simulink model "prelab5"  (R2023b)
settings: Solver=VariableStepAuto  StartTime=0.0  StopTime=2  RelTol=1e-3
undefined symbols (not defined in the file): magnitude
libraries: dspfdesign x2, commsynccomp2 x1
settings Model: Creator=ASUS  LastModifiedBy=ASUS

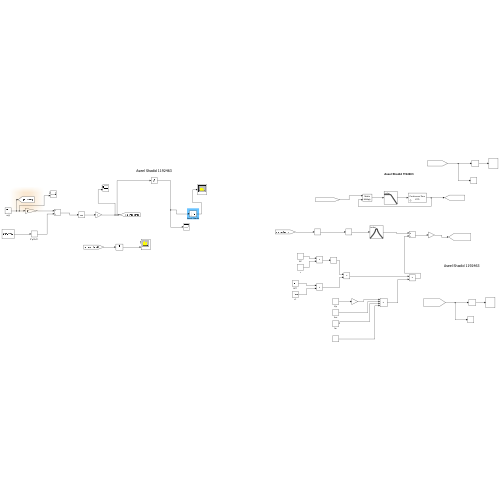
[thumbnail: Simulink's stored preview of the top-level diagram]
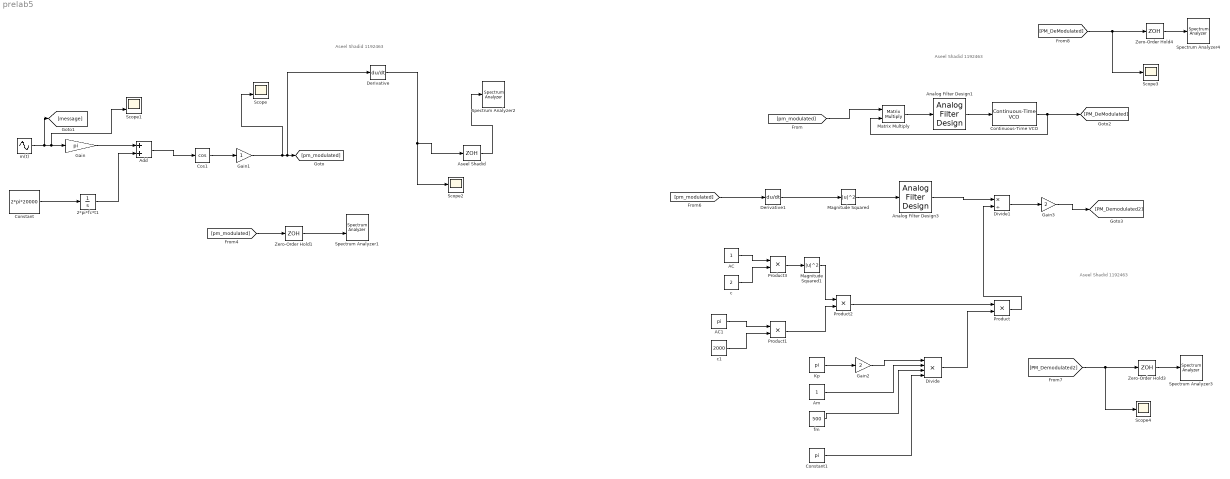
== system prelab5 ==
  note: Aseel Shadid 1192463
  note: Aseel Shadid 1192463
  note: Aseel Shadid 1192463
  " m(t)" : Sin  Frequency=500*pi*2  SampleTime=0
  2*pi*fc*t1 : Integrator
  AC : Constant
  AC1 : Constant  Value=pi
  Add : Sum
  Am : Constant
  Analog Filter Design1 : dspfdesign/Analog Filter Design  method=Butterworth  filttype=Lowpass  N=8  Wlo=pi*2*1000  Whi=80  Rp=2  Rs=40
  Analog Filter Design3 : dspfdesign/Analog Filter Design  method=Butterworth  filttype=Bandpass  N=8  Wlo=pi*2*400  Whi=pi*2*600  Rp=2  Rs=40
  Aseel Shadid : ZeroOrderHold  SampleTime=1/(10*20000)
  Constant : Constant  Value=2*pi*20000
  Constant1 : Constant  Value=pi
  Continuous-Time VCO : commsynccomp2/Continuous-Time VCO  Ac=1  Fc=400  Kc=1  Ph=0
  Cos1 : Trigonometry  Operator=cos
  Derivative : Derivative
  Derivative1 : Derivative
  Divide : Product  Inputs=****
  Divide1 : Product  Inputs=*/
  Gain : Gain  Gain=pi
  Gain1 : Gain
  Gain2 : Gain  Gain=2
  Gain3 : Gain  Gain=2
  Kp : Constant  Value=pi
  Magnitude Squared : Math  Operator=magnitude^2
  Magnitude Squared1 : Math  Operator=magnitude^2
  Matrix Multiply : Product  Multiplication=Matrix(*)
  Product{,1..3} (4 alike) : Product
  Scope : Scope  NumInputPorts=2
  Scope1 : Scope  NumInputPorts=2
  Scope2 : Scope
  Scope3 : Scope
  Scope4 : Scope
  Spectrum Analyzer1 : SpectrumAnalyzer  NumInputPorts=2  WindowPosition=[151.000000,138.000000,1280.000000,605.000000,]  ScopeFrameLocation=window  SpectrumType=RMS  Method=Welch  SampleRate=200000  AxesScaling=Manual  Span=200000  StartFrequency=-100000  StopFrequency=100000  AveragingMethod=Running  SpectrumUnits=Vrms  YLimits=[-0.059214814457474507225,0.53293338124662115174]  DefaultConfigurationName=spbscopes.SpectrumAnalyzerBlockCfg  IsFrequencyInputMode=0  FrequencyVectorPort=0  FrequencyVectorFromPort=0  FrequencyInputRBWPort=0  FrequencyInputRBWFromPort=0
  Spectrum Analyzer2 : SpectrumAnalyzer  WindowPosition=[99.000000,50.000000,1280.000000,605.000000,]  ScopeFrameLocation=window  SpectrumType=RMS  Method=Welch  SampleRate=200000  AxesScaling=Manual  Span=200000  StartFrequency=-100000  StopFrequency=100000  AveragingMethod=Running  SpectrumUnits=Vrms  YLimits=[-3722.990102194120027,33506.911157803537208]  DefaultConfigurationName=spbscopes.SpectrumAnalyzerBlockCfg  IsFrequencyInputMode=0  FrequencyVectorPort=0  FrequencyVectorFromPort=0  FrequencyInputRBWPort=0  FrequencyInputRBWFromPort=0
  Spectrum Analyzer3 : SpectrumAnalyzer  WindowPosition=[15.000000,87.000000,1280.000000,605.000000,]  ScopeFrameLocation=window  SpectrumType=RMS  Method=Welch  SampleRate=200000  AxesScaling=Manual  Span=199999.99999999997  StartFrequency=-99999.99999999999  StopFrequency=99999.99999999999  AveragingMethod=Running  SpectrumUnits=Vrms  YLimits=[-0.54752572772996410677,4.9277315678643134333]  DefaultConfigurationName=spbscopes.SpectrumAnalyzerBlockCfg  IsFrequencyInputMode=0  FrequencyVectorPort=0  FrequencyVectorFromPort=0  FrequencyInputRBWPort=0  FrequencyInputRBWFromPort=0
  Spectrum Analyzer4 : SpectrumAnalyzer  WindowPosition=[-1.000000,139.000000,1280.000000,605.000000,]  ScopeFrameLocation=window  SpectrumType=RMS  Method=Welch  SampleRate=200000  AxesScaling=Manual  Span=200000  StartFrequency=-100000  StopFrequency=100000  AveragingMethod=Running  SpectrumUnits=Vrms  YLimits=[-0.06230515778296413093,0.56074642006213926138]  DefaultConfigurationName=spbscopes.SpectrumAnalyzerBlockCfg  IsFrequencyInputMode=0  FrequencyVectorPort=0  FrequencyVectorFromPort=0  FrequencyInputRBWPort=0  FrequencyInputRBWFromPort=0
  Zero-Order Hold1 : ZeroOrderHold  SampleTime=1/(10*20000)
  Zero-Order Hold3 : ZeroOrderHold  SampleTime=1/(10*20000)
  Zero-Order Hold4 : ZeroOrderHold  SampleTime=1/(10*20000)
  c : Constant  Value=2
  c1 : Constant  Value=2000
  fm : Constant  Value=500
  wires:
  Add/1 -> Cos1/1
  " m(t)"/1 -> [message], Scope1/2, Gain/1
  Gain/1 -> Add/1
  2*pi*fc*t1/1 -> Add/2
  Gain1/1 -> Scope/2, Derivative/1, [pm_modulated]
  Constant/1 -> 2*pi*fc*t1/1
  Cos1/1 -> Gain1/1
  [pm_modulated] -> Zero-Order Hold1/1
  Zero-Order Hold1/1 -> Spectrum Analyzer1/2
  Derivative/1 -> Scope2/1, Aseel Shadid/1
  Aseel Shadid/1 -> Spectrum Analyzer2/1
  [PM_Demodulated2] -> Zero-Order Hold3/1, Scope4/1
  Product/1 -> Divide1/2
  fm/1 -> Divide/3
  c1/1 -> Product1/2
  c/1 -> Product3/2
  Divide/1 -> Product/2
  Product1/1 -> Product2/2
  Am/1 -> Divide/2
  Product2/1 -> Product/1
  Product3/1 -> Magnitude Squared1/1
  Zero-Order Hold3/1 -> Spectrum Analyzer3/1
  Analog Filter Design3/1 -> Divide1/1
  Kp/1 -> Gain2/1
  Gain2/1 -> Divide/1
  Magnitude Squared/1 -> Analog Filter Design3/1
  Divide1/1 -> Gain3/1
  AC/1 -> Product3/1
  AC1/1 -> Product1/1
  [pm_modulated] -> Derivative1/1
  Derivative1/1 -> Magnitude Squared/1
  Gain3/1 -> [PM_Demodulated2]
  Magnitude Squared1/1 -> Product2/1
  Constant1/1 -> Divide/4
  Continuous-Time VCO/1 -> [PM_DeModulated], Matrix Multiply/2
  Matrix Multiply/1 -> Analog Filter Design1/1
  Analog Filter Design1/1 -> Continuous-Time VCO/1
  [PM_DeModulated] -> Zero-Order Hold4/1, Scope3/1
  Zero-Order Hold4/1 -> Spectrum Analyzer4/1
  [pm_modulated] -> Matrix Multiply/1
